simulink model "SpringPendulum"  (R2024a)
settings: Solver=VariableStepAuto  StartTime=0.0  StopTime=10  MaxStep=1e-3  RelTol=1e-3
settings Model: Creator=perruquetti  LastModifiedBy=perruquetti

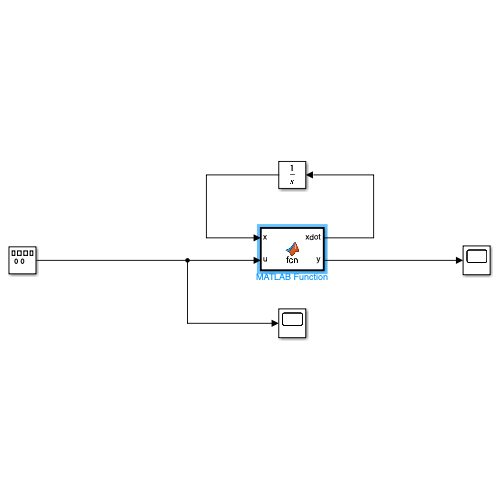
[thumbnail: Simulink's stored preview of the top-level diagram]
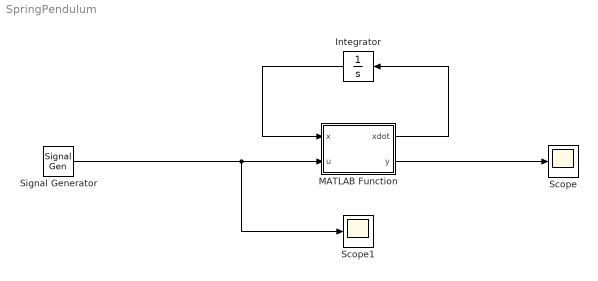
== system SpringPendulum ==
  Integrator : Integrator  InitialCondition="[0.1;  0; 0.84; 0]"
  MATLAB Function : MATLAB Function  TreatAsAtomicUnit=on
  Scope : Scope
  Scope1 : Scope
  Signal Generator : SignalGenerator  Amplitude=0  Frequency=10  Units=rad/sec
  wires:
  MATLAB Function/1(xdot) -> Integrator/1
  Integrator/1 -> MATLAB Function/1(x)
  MATLAB Function/2(y) -> Scope/1
  Signal Generator/1 -> Scope1/1, MATLAB Function/2(u)

== matlab function SpringPendulum/MATLAB Function ==
  data: x input; xdot output; u input; y output
function [xdot,y] = fcn(x,u)
% m \ddot x-2m (\ell+x) {\dot \theta}^2 &=&  mg\cos(\theta) -kx ,\label{eq:Spring pendulum1}\\
% m (\ell+x)^2 \ddot  \theta + 2m (\ell+x) \dot x \dot \theta &=& u+mg
% constants
    m = 0.1; 
    l = 0.1;
    k = 1;
    g = 9.81;

% nonlinear set of equations
    xdot = [x(2);
        2*(l+x(1))*x(4)*x(4)+g*cos(x(3))-k*x(1)/m;
        x(4);
        (u(1)+m*g-2*m*(l+x(1))*x(2)*x(4))/(m*(l+x(1))^2)];
    y = x';
